simulink model "Simulink_task1"  (R2023a)
settings: Solver=VariableStepAuto  StartTime=0.0  StopTime=10.0  RelTol=1e-3
settings Model: Creator=MUHAMMAD SADEEQ  LastModifiedBy=MUHAMMAD SADEEQ

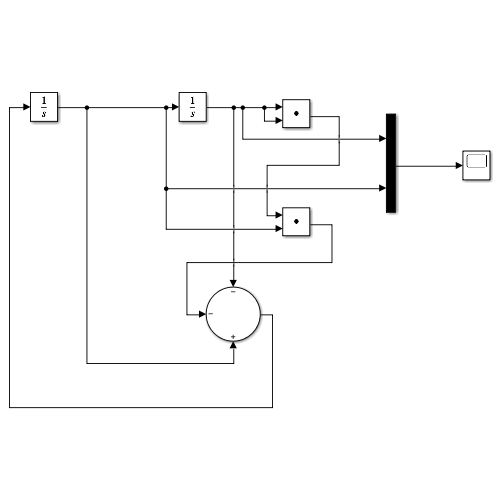
[thumbnail: Simulink's stored preview of the top-level diagram]
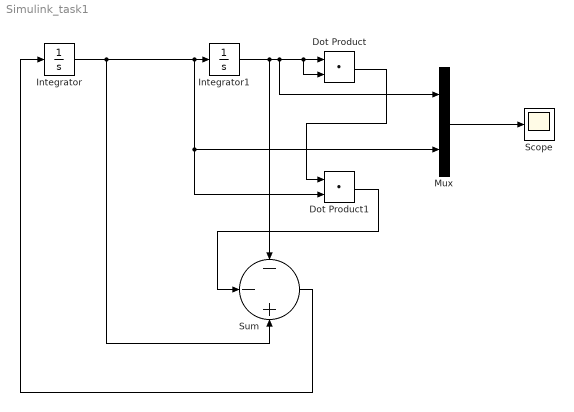
== system Simulink_task1 ==
  Dot Product : DotProduct  OutDataTypeStr=Inherit: Inherit via internal rule
  Dot Product1 : DotProduct  OutDataTypeStr=Inherit: Inherit via internal rule
  Integrator : Integrator  InitialCondition=1
  Integrator1 : Integrator  InitialCondition=2
  Mux : Mux  Inputs=2
  Scope : Scope
  Sum : Sum  Inputs=--+
  wires:
  Integrator/1 -> Dot Product1/2, Mux/2, Integrator1/1, Sum/3
  Integrator1/1 -> Mux/1, Dot Product/2, Dot Product/1, Sum/1
  Mux/1 -> Scope/1
  Dot Product/1 -> Dot Product1/1
  Sum/1 -> Integrator/1
  Dot Product1/1 -> Sum/2
